simulink model "consensus_swarm_3"  (R2026a)
settings: Solver=ode4  FixedStep=0.004
undefined symbols (not defined in the file or in its folder): consensus_swarm_step, controlParams, eQ, eT, GravityAcc, kQ, kT, Mass, minPWM, rotorsSpeedDown, rotorsSpeedUp, SampleTime, uavParam
libraries: slpidlib x72, simulink x33, robotcorelib x12, matrix_library x12, aerolibasang x12, aerolibobsolete x3, uavutilslib x3
(part 1 of 9)
settings Model: Creator=Aaron  LastModifiedBy=Aaron

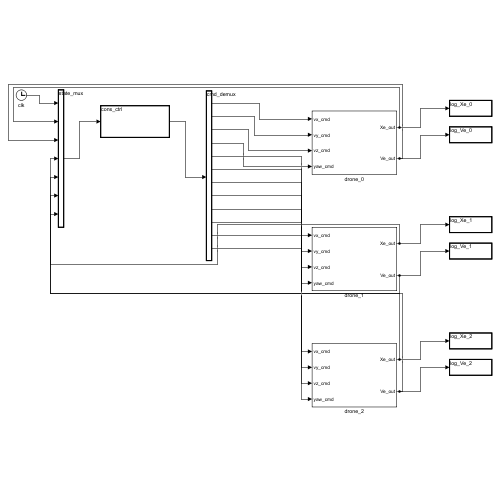
[thumbnail: Simulink's stored preview of the top-level diagram]
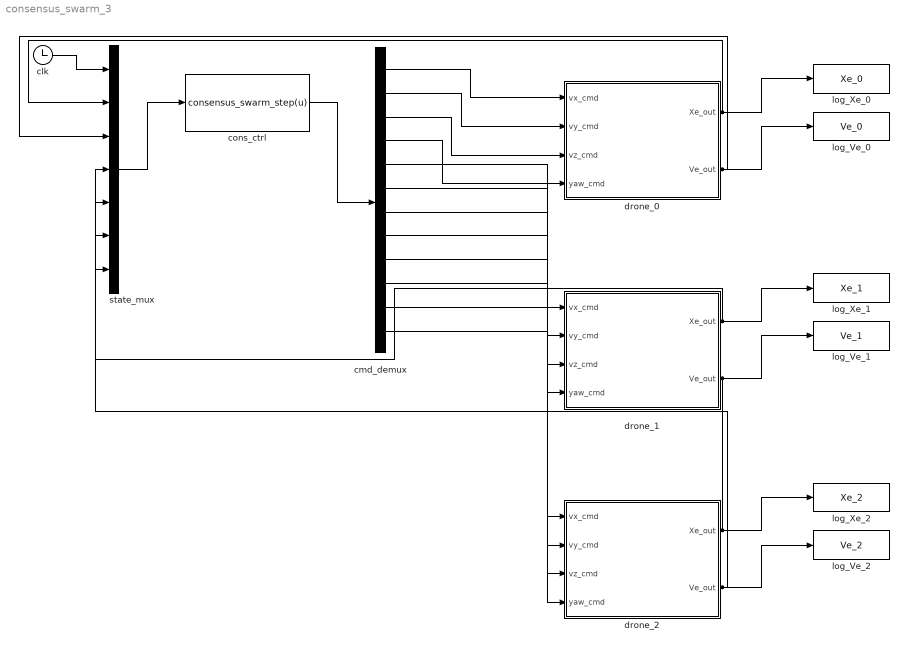
== system consensus_swarm_3 ==
  clk : Clock
  cmd_demux : Demux  Outputs=12
  cons_ctrl : MATLABFcn  MATLABFcn=consensus_swarm_step(u)  OutputDimensions=12  SampleTime=0.02
  drone_0 : Subsystem
  drone_1 : Subsystem
  drone_2 : Subsystem
  log_Ve_0 : ToWorkspace  VariableName=Ve_0  SaveFormat=Timeseries  SampleTime=-1
  log_Ve_1 : ToWorkspace  VariableName=Ve_1  SaveFormat=Timeseries  SampleTime=-1
  log_Ve_2 : ToWorkspace  VariableName=Ve_2  SaveFormat=Timeseries  SampleTime=-1
  log_Xe_0 : ToWorkspace  VariableName=Xe_0  SaveFormat=Timeseries  SampleTime=-1
  log_Xe_1 : ToWorkspace  VariableName=Xe_1  SaveFormat=Timeseries  SampleTime=-1
  log_Xe_2 : ToWorkspace  VariableName=Xe_2  SaveFormat=Timeseries  SampleTime=-1
  state_mux : Mux  Inputs=7
  wires:
  clk/1 -> state_mux/1
  state_mux/1 -> cons_ctrl/1
  cons_ctrl/1 -> cmd_demux/1
  drone_0/1(Xe_out) -> state_mux/2, log_Xe_0/1
  drone_0/2(Ve_out) -> state_mux/3, log_Ve_0/1
  cmd_demux/1 -> drone_0/1(vx_cmd)
  cmd_demux/2 -> drone_0/2(vy_cmd)
  cmd_demux/3 -> drone_0/3(vz_cmd)
  cmd_demux/4 -> drone_0/4(yaw_cmd)
  drone_1/1(Xe_out) -> state_mux/4, log_Xe_1/1
  drone_1/2(Ve_out) -> state_mux/5, log_Ve_1/1
  cmd_demux/5 -> drone_1/1(vx_cmd)
  cmd_demux/6 -> drone_1/2(vy_cmd)
  cmd_demux/7 -> drone_1/3(vz_cmd)
  cmd_demux/8 -> drone_1/4(yaw_cmd)
  drone_2/1(Xe_out) -> state_mux/6, log_Xe_2/1
  drone_2/2(Ve_out) -> state_mux/7, log_Ve_2/1
  cmd_demux/9 -> drone_2/1(vx_cmd)
  cmd_demux/10 -> drone_2/2(vy_cmd)
  cmd_demux/11 -> drone_2/3(vz_cmd)
  cmd_demux/12 -> drone_2/4(yaw_cmd)

== system consensus_swarm_3/drone_0 ==
  vx_cmd : Inport
  vy_cmd : Inport  Port=2
  vz_cmd : Inport  Port=3
  yaw_cmd : Inport  Port=4
  6DOF (Euler Angles) : aerolibobsolete/6DOF (Euler Angles)  units=Metric (MKS)  mtype=Fixed  rep=Euler Angles  xme_0=[0, 0, 0]  Vm_0=[0 0 0]  eul_0=[0 0 0]  pm_0=[0 0 0]  mass_0=Mass  mass_e=0.5  mass_f=2.0  inertia=momentInertia  inertia_e=eye(3)  inertia_f=2*eye(3)  k_quat=1.0  vre_flag=on  abi_flag=on  aMode=0  xme_statename=''  Vm_statename=''  eul_statename=''  quat_statename=''  pm_statename=''  mass_statename=''
  Add : Sum
  Bus Creator : BusCreator  Inputs=4
  Display17 : Display
  Gravity : Subsystem
  Mux4 : Mux  Inputs=3
  Selector1 : Selector  InputPortWidth=3  IndexOptions=Index vector (dialog)  Indices=[3 2 1]  OutputSizes=1
  Step4 : Step  Time=5  SampleTime=0
  Subsystem : Subsystem
  UAV Animation : uavutilslib/UAV Animation  Commented=on  NumUAV=1  DynamicUAVConfig=off  UAVType=Multirotor  UAVSize=5  UAVColor=[1 0 0]  UAVTrajectoryAlpha=1  AlwaysShowAnimation=on  AxisLimits=[-Inf Inf;-Inf Inf;-Inf Inf]  TrajectoryBufferSize=100000  InertialZDirection=Down  RotationFormat=Euler ZYX  DrawMarkers=off  SampleTime=-1
  pid_velocity : Subsystem
  z : Constant  Value=0
  Xe_out : Outport
  Ve_out : Outport  Port=2
  wires:
  Mux4/1 -> pid_velocity/2(vxyz_d)  "vel_cmd"
  z/1 -> ?
  [States] -> pid_velocity/1(estStates)
  pid_velocity/1(acts_w) -> Display17/1, [pid_pos]  "pid"
  [pid_pos] -> Subsystem/1(actCmd)
  Add/1 -> 6DOF (Euler Angles)/1
  Subsystem/1(F) -> Add/1
  Gravity/1(F_g) -> Add/2  "Gravity Force"
  Subsystem/2(M) -> 6DOF (Euler Angles)/2
  Bus Creator/1 -> [States]
  6DOF (Euler Angles)/4 -> [DCMbe]  "DCMbe"
  [DCMbe] -> Gravity/1(DCM_be)
  6DOF (Euler Angles)/1 -> Ve_out/1, [Ve]  "Ve"
  [Ve] -> Bus Creator/1
  [Xe] -> Bus Creator/2
  6DOF (Euler Angles)/3 -> [Euler], Selector1/1  "Euler"
  [Euler] -> Bus Creator/3
  6DOF (Euler Angles)/6 -> [pqr]  "pqr"
  [pqr] -> Bus Creator/4
  6DOF (Euler Angles)/2 -> Xe_out/1, [Xe], UAV Animation/1  "Xe"
  Selector1/1 -> UAV Animation/2
  vx_cmd/1 -> Mux4/1
  vy_cmd/1 -> Mux4/2
  vz_cmd/1 -> Mux4/3
  yaw_cmd/1 -> [uav_plant_io_yaw_cmd]

== system consensus_swarm_3/drone_1 ==
  vx_cmd : Inport
  vy_cmd : Inport  Port=2
  vz_cmd : Inport  Port=3
  yaw_cmd : Inport  Port=4
  6DOF (Euler Angles) : aerolibobsolete/6DOF (Euler Angles)  units=Metric (MKS)  mtype=Fixed  rep=Euler Angles  xme_0=[0, 0, 0]  Vm_0=[0 0 0]  eul_0=[0 0 0]  pm_0=[0 0 0]  mass_0=Mass  mass_e=0.5  mass_f=2.0  inertia=momentInertia  inertia_e=eye(3)  inertia_f=2*eye(3)  k_quat=1.0  vre_flag=on  abi_flag=on  aMode=0  xme_statename=''  Vm_statename=''  eul_statename=''  quat_statename=''  pm_statename=''  mass_statename=''
  Add : Sum
  Bus Creator : BusCreator  Inputs=4
  Display17 : Display
  Gravity : Subsystem
  Mux4 : Mux  Inputs=3
  Selector1 : Selector  InputPortWidth=3  IndexOptions=Index vector (dialog)  Indices=[3 2 1]  OutputSizes=1
  Step4 : Step  Time=5  SampleTime=0
  Subsystem : Subsystem
  UAV Animation : uavutilslib/UAV Animation  Commented=on  NumUAV=1  DynamicUAVConfig=off  UAVType=Multirotor  UAVSize=5  UAVColor=[1 0 0]  UAVTrajectoryAlpha=1  AlwaysShowAnimation=on  AxisLimits=[-Inf Inf;-Inf Inf;-Inf Inf]  TrajectoryBufferSize=100000  InertialZDirection=Down  RotationFormat=Euler ZYX  DrawMarkers=off  SampleTime=-1
  pid_velocity : Subsystem
  z : Constant  Value=0
  Xe_out : Outport
  Ve_out : Outport  Port=2
  wires:
  Mux4/1 -> pid_velocity/2(vxyz_d)  "vel_cmd"
  z/1 -> ?
  [States] -> pid_velocity/1(estStates)
  pid_velocity/1(acts_w) -> Display17/1, [pid_pos]  "pid"
  [pid_pos] -> Subsystem/1(actCmd)
  Add/1 -> 6DOF (Euler Angles)/1
  Subsystem/1(F) -> Add/1
  Gravity/1(F_g) -> Add/2  "Gravity Force"
  Subsystem/2(M) -> 6DOF (Euler Angles)/2
  Bus Creator/1 -> [States]
  6DOF (Euler Angles)/4 -> [DCMbe]  "DCMbe"
  [DCMbe] -> Gravity/1(DCM_be)
  6DOF (Euler Angles)/1 -> Ve_out/1, [Ve]  "Ve"
  [Ve] -> Bus Creator/1
  [Xe] -> Bus Creator/2
  6DOF (Euler Angles)/3 -> [Euler], Selector1/1  "Euler"
  [Euler] -> Bus Creator/3
  6DOF (Euler Angles)/6 -> [pqr]  "pqr"
  [pqr] -> Bus Creator/4
  6DOF (Euler Angles)/2 -> Xe_out/1, [Xe], UAV Animation/1  "Xe"
  Selector1/1 -> UAV Animation/2
  vx_cmd/1 -> Mux4/1
  vy_cmd/1 -> Mux4/2
  vz_cmd/1 -> Mux4/3
  yaw_cmd/1 -> [uav_plant_io_yaw_cmd]

== system consensus_swarm_3/drone_2 ==
  vx_cmd : Inport
  vy_cmd : Inport  Port=2
  vz_cmd : Inport  Port=3
  yaw_cmd : Inport  Port=4
  6DOF (Euler Angles) : aerolibobsolete/6DOF (Euler Angles)  units=Metric (MKS)  mtype=Fixed  rep=Euler Angles  xme_0=[0, 0, 0]  Vm_0=[0 0 0]  eul_0=[0 0 0]  pm_0=[0 0 0]  mass_0=Mass  mass_e=0.5  mass_f=2.0  inertia=momentInertia  inertia_e=eye(3)  inertia_f=2*eye(3)  k_quat=1.0  vre_flag=on  abi_flag=on  aMode=0  xme_statename=''  Vm_statename=''  eul_statename=''  quat_statename=''  pm_statename=''  mass_statename=''
  Add : Sum
  Bus Creator : BusCreator  Inputs=4
  Display17 : Display
  Gravity : Subsystem
  Mux4 : Mux  Inputs=3
  Selector1 : Selector  InputPortWidth=3  IndexOptions=Index vector (dialog)  Indices=[3 2 1]  OutputSizes=1
  Step4 : Step  Time=5  SampleTime=0
  Subsystem : Subsystem
  UAV Animation : uavutilslib/UAV Animation  Commented=on  NumUAV=1  DynamicUAVConfig=off  UAVType=Multirotor  UAVSize=5  UAVColor=[1 0 0]  UAVTrajectoryAlpha=1  AlwaysShowAnimation=on  AxisLimits=[-Inf Inf;-Inf Inf;-Inf Inf]  TrajectoryBufferSize=100000  InertialZDirection=Down  RotationFormat=Euler ZYX  DrawMarkers=off  SampleTime=-1
  pid_velocity : Subsystem
  z : Constant  Value=0
  Xe_out : Outport
  Ve_out : Outport  Port=2
  wires:
  Mux4/1 -> pid_velocity/2(vxyz_d)  "vel_cmd"
  z/1 -> ?
  [States] -> pid_velocity/1(estStates)
  pid_velocity/1(acts_w) -> Display17/1, [pid_pos]  "pid"
  [pid_pos] -> Subsystem/1(actCmd)
  Add/1 -> 6DOF (Euler Angles)/1
  Subsystem/1(F) -> Add/1
  Gravity/1(F_g) -> Add/2  "Gravity Force"
  Subsystem/2(M) -> 6DOF (Euler Angles)/2
  Bus Creator/1 -> [States]
  6DOF (Euler Angles)/4 -> [DCMbe]  "DCMbe"
  [DCMbe] -> Gravity/1(DCM_be)
  6DOF (Euler Angles)/1 -> Ve_out/1, [Ve]  "Ve"
  [Ve] -> Bus Creator/1
  [Xe] -> Bus Creator/2
  6DOF (Euler Angles)/3 -> [Euler], Selector1/1  "Euler"
  [Euler] -> Bus Creator/3
  6DOF (Euler Angles)/6 -> [pqr]  "pqr"
  [pqr] -> Bus Creator/4
  6DOF (Euler Angles)/2 -> Xe_out/1, [Xe], UAV Animation/1  "Xe"
  Selector1/1 -> UAV Animation/2
  vx_cmd/1 -> Mux4/1
  vy_cmd/1 -> Mux4/2
  vz_cmd/1 -> Mux4/3
  yaw_cmd/1 -> [uav_plant_io_yaw_cmd]

== system consensus_swarm_3/drone_0/Gravity ==
  DCM_be : Inport
  Constant : Constant  Value=[0 0 GravityAcc]'
  Display4 : Display
  Gain : Gain  Gain=Mass
  Matrix Multiply : Product  Multiplication=Matrix(*)
  F_g : Outport
  wires:
  Gain/1 -> F_g/1, Display4/1
  DCM_be/1 -> Matrix Multiply/1
  Constant/1 -> Matrix Multiply/2
  Matrix Multiply/1 -> Gain/1

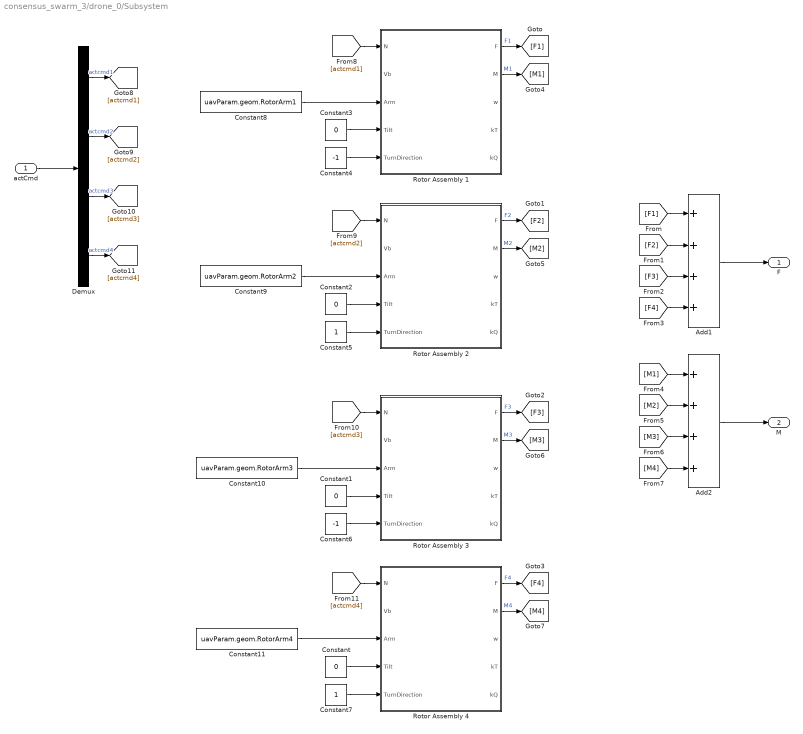
== system consensus_swarm_3/drone_0/Subsystem ==
  actCmd : Inport
  Add1 : Sum  Inputs=++++
  Add2 : Sum  Inputs=++++
  Constant{,1..3} (4 alike) : Constant  Value=0
  Constant10 : Constant  Value=uavParam.geom.RotorArm3
  Constant11 : Constant  Value=uavParam.geom.RotorArm4
  Constant4 : Constant  Value=-1
  Constant5 : Constant
  Constant6 : Constant  Value=-1
  Constant7 : Constant
  Constant8 : Constant  Value=uavParam.geom.RotorArm1
  Constant9 : Constant  Value=uavParam.geom.RotorArm2
  Demux : Demux
  Rotor Assembly 1 : Subsystem
  Rotor Assembly 2 : Subsystem
  Rotor Assembly 3 : Subsystem
  Rotor Assembly 4 : Subsystem
  F : Outport
  M : Outport  Port=2
  wires:
  [actcmd4] -> Rotor Assembly 4/1(N)
  Demux/4 -> [actcmd4]  "actcmd4"
  [actcmd3] -> Rotor Assembly 3/1(N)
  Demux/3 -> [actcmd3]  "actcmd3"
  [actcmd2] -> Rotor Assembly 2/1(N)
  Demux/2 -> [actcmd2]  "actcmd2"
  [actcmd1] -> Rotor Assembly 1/1(N)
  Demux/1 -> [actcmd1]  "actcmd1"
  actCmd/1 -> Demux/1
  [M4] -> Add2/4
  Rotor Assembly 4/2(M) -> [M4]  "M4"
  [M3] -> Add2/3
  Rotor Assembly 3/2(M) -> [M3]  "M3"
  [M2] -> Add2/2
  Rotor Assembly 2/2(M) -> [M2]  "M2"
  [M1] -> Add2/1
  Rotor Assembly 1/2(M) -> [M1]  "M1"
  [F4] -> Add1/4
  Rotor Assembly 4/1(F) -> [F4]  "F4"
  [F3] -> Add1/3
  Rotor Assembly 3/1(F) -> [F3]  "F3"
  [F2] -> Add1/2
  Rotor Assembly 2/1(F) -> [F2]  "F2"
  [F1] -> Add1/1
  Rotor Assembly 1/1(F) -> [F1]  "F1"
  Constant11/1 -> Rotor Assembly 4/3(Arm)
  Constant9/1 -> Rotor Assembly 2/3(Arm)
  Constant8/1 -> Rotor Assembly 1/3(Arm)
  Constant7/1 -> Rotor Assembly 4/5(TurnDirection)
  Constant5/1 -> Rotor Assembly 2/5(TurnDirection)
  Constant4/1 -> Rotor Assembly 1/5(TurnDirection)
  Constant3/1 -> Rotor Assembly 1/4(Tilt)
  Constant2/1 -> Rotor Assembly 2/4(Tilt)
  Constant/1 -> Rotor Assembly 4/4(Tilt)
  Add2/1 -> M/1
  Constant1/1 -> Rotor Assembly 3/4(Tilt)
  Constant6/1 -> Rotor Assembly 3/5(TurnDirection)
  ? -> Rotor Assembly 3/2(Vb)
  Add1/1 -> F/1
  Constant10/1 -> Rotor Assembly 3/3(Arm)

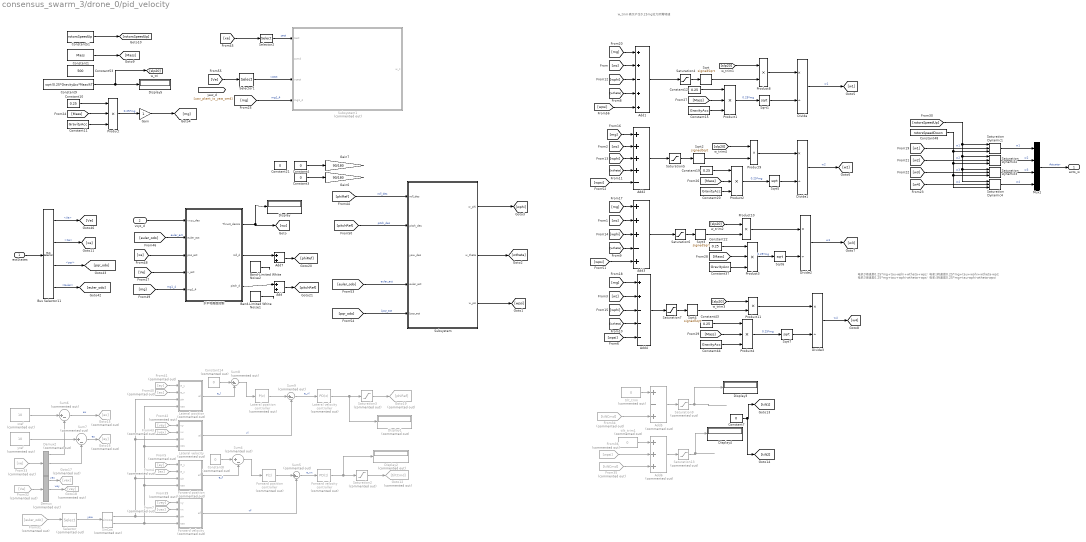
== system consensus_swarm_3/drone_0/pid_velocity ==
  note: w_trim 表示产生0.25mg拉力所需转速
  note: 电机1转速是0.25*mg+tau-wphi+wtheta+wpsi，
      | 电机2转速是0.25*mg+tau+wphi+wtheta-wpsi，
      | 电机3转速是0.25*mg+tau+wphi-wtheta+wpsi，
      | 电机4转速是0.25*mg+tau-wphi-wtheta-wpsi
  estStates : Inport
  vxyz_d : Inport  Port=2
  Add : Sum
  Add1 : Sum  Inputs=++-++
  Add2 : Sum  Inputs=++++-
  Add3 : Sum  Inputs=+++-+
  Add4 : Sum  Inputs=++---
  Add5 : Sum  Commented=on  Inputs=+-+
  Add6 : Sum  Commented=on  Inputs=+++
  Add7 : Sum
  Band-Limited White Noise1 : simulink/Sources/Band-Limited White Noise  Cov=[0.000001]  Ts=SampleTime  seed=[23341]
  Band-Limited White Noise2 : simulink/Sources/Band-Limited White Noise  Cov=[0.000001]  Ts=SampleTime  seed=[2341]
  Bus Selector11 : BusSelector  OutputSignals=Ve,Xe,pqr,Euler
  Constant1 : Constant  Value=Mass  OutDataTypeStr=double
  Constant{10,12,19,22,43} (5 alike) : Constant  Value=0.25  OutDataTypeStr=double
  Constant{11,15,20,37,44} (5 alike) : Constant  Value=GravityAcc  OutDataTypeStr=double
  Constant14 : Constant  Commented=on  Value=0
  Constant{3..4,7,21} (4 alike) : Constant  Value=0  OutDataTypeStr=double
  Constant48 : Constant  Value=rotorsSpeedDown  OutDataTypeStr=double
  Constant51 : Constant  Value=rotorsSpeedUp  OutDataTypeStr=double
  Constant53 : Constant  Value=500
  Constant8 : Constant  Commented=on  Value=0
  Constant9 : Constant  Value=sqrt(0.25*GravityAcc*Mass/kT)
  Demux : Demux  Commented=on  Outputs=3
  Demux2 : Demux  Commented=on  Outputs=3
  Display{,3..5} (4 alike) : Display
  Display1 : Display  Commented=on
  Display2 : Display  Commented=on
  Divide{,1..3} (4 alike) : Product  Inputs=*/
  Forward position : Subsystem  Commented=on
  Forward position controller : slpidlib/PID Controller  Commented=on  Controller=P  Form=Parallel  TimeDomain=Discrete-time  UseExternalTs=off  SampleTime=-1  IntegratorMethod=Forward Euler  FilterMethod=Forward Euler  ControllerParametersSource=internal  P=1  I=controlParams.I_X  UseKiTs=off  D=0.741088334151374  UseExternalDerivativeSource=off  N=1.14081860742283  UseFilter=on  TunerSelectOption=Transfer Function Based (PID Tuner App)  InitialConditionSource=internal  InitialConditionForIntegrator=0  InitialConditionForFilter=0  DifferentiatorICPrevScaledInput=0  ExternalReset=none  TrackingMode=off  Kt=1  LimitOutput=off  SatLimitsSource=internal  UpperSaturationLimit=inf  LowerSaturationLimit=-inf  LinearizeAsGain=on  AntiWindupMode=none  Kb=1  LimitIntegrator=off  UpperIntegratorSaturationLimit=inf  LowerIntegratorSaturationLimit=-inf  POutMin=[]  POutMax=[]  IOutMin=[]  IOutMax=[]  DOutMin=[]  DOutMax=[]  NOutMin=[]  NOutMax=[]  SumOutMin=[]  SumOutMax=[]  SaturationOutMin=[]  SaturationOutMax=[]  PParamMin=[]  PParamMax=[]  IParamMin=[]  IParamMax=[]  DParamMin=[]  DParamMax=[]  NParamMin=[]  NParamMax=[]  KbParamMin=[]  KbParamMax=[]  KtParamMin=[]  KtParamMax=[]  KbOutMin=[]  KbOutMax=[]  KtOutMin=[]  KtOutMax=[]  IntegratorOutMin=[]  IntegratorOutMax=[]  FilterOutMin=[]  FilterOutMax=[]  SumI1OutMin=[]  SumI1OutMax=[]  SumI2OutMin=[]  SumI2OutMax=[]  SumI3OutMin=[]  SumI3OutMax=[]  SumI4OutMin=[]  SumI4OutMax=[]  SumDOutMin=[]  SumDOutMax=[]  DifferentiatorOutMin=[]  DifferentiatorOutMax=[]  FilterDiffOutCoefMin=[]  FilterDiffOutCoefMax=[]  ReciprocalOutMin=[]  ReciprocalOutMax=[]  SumDenOutMin=[]  SumDenOutMax=[]  SumNumOutMin=[]  SumNumOutMax=[]  DivideOutMin=[]  DivideOutMax=[]  UdiffTsProdOutMin=[]  UdiffTsProdOutMax=[]  NTsProdOutMin=[]  NTsProdOutMax=[]  UintegralTsProdOutMin=[]  UintegralTsProdOutMax=[]  UngainTsProdOutMin=[]  UngainTsProdOutMax=[]  ClampingZeroOutDataTypeStr=Inherit: Inherit via back propagation  ClampingZeroOutMin=[]  ClampingZeroOutMax=[]  FilterDenConstantOutDataTypeStr=Inherit: Inherit via back propagation  FilterDenConstantOutMin=[]  FilterDenConstantOutMax=[]  PCopyOutDataTypeStr=Inherit: Inherit via back propagation  PCopyOutMin=[]  PCopyOutMax=[]  NCopyOutDataTypeStr=Inherit: Inherit via back propagation  NCopyOutMin=[]  NCopyOutMax=[]  IntegratorContinuousStateAttributes=''  IntegratorStateMustResolveToSignalObject=off  IntegratorRTWStateStorageClass=Auto  FilterContinuousStateAttributes=''  FilterStateMustResolveToSignalObject=off  FilterRTWStateStorageClass=Auto  ParallelPVariant=InternalParameters  IdealPVariant=Disabled  IVariant=Disabled  DVariant=Disabled  IntegratorVariant=Disabled  SatVariant=Disabled  AWVariant=Disabled  PCopyVariant=Disabled  TRVariant=Disabled  FdbkBlocksVariant=Forward  IdealPFdbkVariant=Disabled  SatFdbkVariant=Disabled  DerivativeFilterVariant=Disabled  NVariant=Disabled  NCopyVariant=Disabled_SignalSpec  FilterICVariant=Disabled  IntegratorICVariant=Disabled  ExternalResetVariant=Disabled  TRSumVariant=Passthrough  SumFdbkVariant=Disabled  SumVariant=Passthrough_P  TsampFilterVariant=InternalTs  TsampNgainVariant=Passthrough  TsampIntegralVariant=Disabled_SignalSpec  ExternalSaturationOutDataTypeStr=Inherit: Same as second input  DerivativeSourceVariant=Disabled  PreIntVariant=InternalPreInt
  Forward velocity : Subsystem  Commented=on
  Forward velocity controller : slpidlib/PID Controller  Commented=on  Controller=PD  Form=Parallel  TimeDomain=Discrete-time  UseExternalTs=off  SampleTime=-1  IntegratorMethod=Forward Euler  FilterMethod=Forward Euler  ControllerParametersSource=internal  P=10  I=0  UseKiTs=off  D=0.1  UseExternalDerivativeSource=off  N=20  UseFilter=on  TunerSelectOption=Transfer Function Based (PID Tuner App)  InitialConditionSource=internal  InitialConditionForIntegrator=0  InitialConditionForFilter=0  DifferentiatorICPrevScaledInput=0  ExternalReset=none  TrackingMode=off  Kt=1  LimitOutput=off  SatLimitsSource=internal  UpperSaturationLimit=inf  LowerSaturationLimit=-inf  LinearizeAsGain=on  AntiWindupMode=none  Kb=1  LimitIntegrator=off  UpperIntegratorSaturationLimit=inf  LowerIntegratorSaturationLimit=-inf  POutMin=[]  POutMax=[]  IOutMin=[]  IOutMax=[]  DOutMin=[]  DOutMax=[]  NOutMin=[]  NOutMax=[]  SumOutMin=[]  SumOutMax=[]  SaturationOutMin=[]  SaturationOutMax=[]  PParamMin=[]  PParamMax=[]  IParamMin=[]  IParamMax=[]  DParamMin=[]  DParamMax=[]  NParamMin=[]  NParamMax=[]  KbParamMin=[]  KbParamMax=[]  KtParamMin=[]  KtParamMax=[]  KbOutMin=[]  KbOutMax=[]  KtOutMin=[]  KtOutMax=[]  IntegratorOutMin=[]  IntegratorOutMax=[]  FilterOutMin=[]  FilterOutMax=[]  SumI1OutMin=[]  SumI1OutMax=[]  SumI2OutMin=[]  SumI2OutMax=[]  SumI3OutMin=[]  SumI3OutMax=[]  SumI4OutMin=[]  SumI4OutMax=[]  SumDOutMin=[]  SumDOutMax=[]  DifferentiatorOutMin=[]  DifferentiatorOutMax=[]  FilterDiffOutCoefMin=[]  FilterDiffOutCoefMax=[]  ReciprocalOutMin=[]  ReciprocalOutMax=[]  SumDenOutMin=[]  SumDenOutMax=[]  SumNumOutMin=[]  SumNumOutMax=[]  DivideOutMin=[]  DivideOutMax=[]  UdiffTsProdOutMin=[]  UdiffTsProdOutMax=[]  NTsProdOutMin=[]  NTsProdOutMax=[]  UintegralTsProdOutMin=[]  UintegralTsProdOutMax=[]  UngainTsProdOutMin=[]  UngainTsProdOutMax=[]  ClampingZeroOutDataTypeStr=Inherit: Inherit via back propagation  ClampingZeroOutMin=[]  ClampingZeroOutMax=[]  FilterDenConstantOutDataTypeStr=Inherit: Inherit via back propagation  FilterDenConstantOutMin=[]  FilterDenConstantOutMax=[]  PCopyOutDataTypeStr=Inherit: Inherit via back propagation  PCopyOutMin=[]  PCopyOutMax=[]  NCopyOutDataTypeStr=Inherit: Inherit via back propagation  NCopyOutMin=[]  NCopyOutMax=[]  IntegratorContinuousStateAttributes=''  IntegratorStateMustResolveToSignalObject=off  IntegratorRTWStateStorageClass=Auto  FilterContinuousStateAttributes=''  FilterStateMustResolveToSignalObject=off  FilterRTWStateStorageClass=Auto  ParallelPVariant=InternalParameters  IdealPVariant=Disabled  IVariant=Disabled  DVariant=InternalParameters  IntegratorVariant=Disabled  SatVariant=Disabled  AWVariant=Disabled  PCopyVariant=Disabled  TRVariant=Disabled  FdbkBlocksVariant=Forward  IdealPFdbkVariant=Disabled  SatFdbkVariant=Disabled  DerivativeFilterVariant=ForwardEulerFilter  NVariant=InternalParameters  NCopyVariant=Disabled  FilterICVariant=InternalICsFilter  IntegratorICVariant=Disabled  ExternalResetVariant=Disabled  TRSumVariant=Passthrough  SumFdbkVariant=Disabled  SumVariant=Sum_PD  TsampFilterVariant=InternalTs  TsampNgainVariant=Passthrough  TsampIntegralVariant=Disabled_SignalSpec  ExternalSaturationOutDataTypeStr=Inherit: Same as second input  DerivativeSourceVariant=ErrorSignal  PreIntVariant=InternalPreInt
  From31 : From  Commented=on  GotoTag=euler_odo
  From32 : From  Commented=on  GotoTag=Ve
  From33 : From  Commented=on  GotoTag=xe
  From34 : From  Commented=on  GotoTag=tiltCmd
  From35 : From  Commented=on  GotoTag=tiltCmd
  From36 : From  Commented=on  GotoTag=wpsi
  From39 : From  Commented=on  GotoTag=vey
  From4 : From  Commented=on  GotoTag=ex
  From40 : From  Commented=on  GotoTag=ex
  From41 : From  Commented=on  GotoTag=ey
  From42 : From  Commented=on  GotoTag=vey
  From43 : From  Commented=on  GotoTag=vex
  From5 : From  Commented=on  GotoTag=ey
  From7 : From  Commented=on  GotoTag=vex
  Gain : Gain
  Gain6 : Gain  Gain=90/180
  Gain7 : Gain  Gain=90/180
  Goto12 : Goto  Commented=on  GotoTag=tiltCmd
  Goto15 : Goto  Commented=on  GotoTag=ex
  Goto16 : Goto  Commented=on  GotoTag=ey
  Goto17 : Goto  Commented=on  GotoTag=vex
  Goto18 : Goto  Commented=on  GotoTag=vey
  Goto19 : Goto  Commented=on  GotoTag=phiRef
  Lateral position : Subsystem  Commented=on
  Lateral position controller : slpidlib/PID Controller  Commented=on  Controller=P  Form=Parallel  TimeDomain=Discrete-time  UseExternalTs=off  SampleTime=-1  IntegratorMethod=Forward Euler  FilterMethod=Forward Euler  ControllerParametersSource=internal  P=1  I=controlParams.I_Y  UseKiTs=off  D=0.20966837124708  UseExternalDerivativeSource=off  N=1.18305565097938  UseFilter=on  TunerSelectOption=Transfer Function Based (PID Tuner App)  InitialConditionSource=internal  InitialConditionForIntegrator=0  InitialConditionForFilter=0  DifferentiatorICPrevScaledInput=0  ExternalReset=none  TrackingMode=off  Kt=1  LimitOutput=off  SatLimitsSource=internal  UpperSaturationLimit=0.4  LowerSaturationLimit=-0.4  LinearizeAsGain=on  AntiWindupMode=clamping  Kb=1  LimitIntegrator=off  UpperIntegratorSaturationLimit=inf  LowerIntegratorSaturationLimit=-inf  POutMin=[]  POutMax=[]  IOutMin=[]  IOutMax=[]  DOutMin=[]  DOutMax=[]  NOutMin=[]  NOutMax=[]  SumOutMin=[]  SumOutMax=[]  SaturationOutMin=[]  SaturationOutMax=[]  PParamMin=[]  PParamMax=[]  IParamMin=[]  IParamMax=[]  DParamMin=[]  DParamMax=[]  NParamMin=[]  NParamMax=[]  KbParamMin=[]  KbParamMax=[]  KtParamMin=[]  KtParamMax=[]  KbOutMin=[]  KbOutMax=[]  KtOutMin=[]  KtOutMax=[]  IntegratorOutMin=[]  IntegratorOutMax=[]  FilterOutMin=[]  FilterOutMax=[]  SumI1OutMin=[]  SumI1OutMax=[]  SumI2OutMin=[]  SumI2OutMax=[]  SumI3OutMin=[]  SumI3OutMax=[]  SumI4OutMin=[]  SumI4OutMax=[]  SumDOutMin=[]  SumDOutMax=[]  DifferentiatorOutMin=[]  DifferentiatorOutMax=[]  FilterDiffOutCoefMin=[]  FilterDiffOutCoefMax=[]  ReciprocalOutMin=[]  ReciprocalOutMax=[]  SumDenOutMin=[]  SumDenOutMax=[]  SumNumOutMin=[]  SumNumOutMax=[]  DivideOutMin=[]  DivideOutMax=[]  UdiffTsProdOutMin=[]  UdiffTsProdOutMax=[]  NTsProdOutMin=[]  NTsProdOutMax=[]  UintegralTsProdOutMin=[]  UintegralTsProdOutMax=[]  UngainTsProdOutMin=[]  UngainTsProdOutMax=[]  ClampingZeroOutDataTypeStr=Inherit: Inherit via back propagation  ClampingZeroOutMin=[]  ClampingZeroOutMax=[]  FilterDenConstantOutDataTypeStr=Inherit: Inherit via back propagation  FilterDenConstantOutMin=[]  FilterDenConstantOutMax=[]  PCopyOutDataTypeStr=Inherit: Inherit via back propagation  PCopyOutMin=[]  PCopyOutMax=[]  NCopyOutDataTypeStr=Inherit: Inherit via back propagation  NCopyOutMin=[]  NCopyOutMax=[]  IntegratorContinuousStateAttributes=''  IntegratorStateMustResolveToSignalObject=off  IntegratorRTWStateStorageClass=Auto  FilterContinuousStateAttributes=''  FilterStateMustResolveToSignalObject=off  FilterRTWStateStorageClass=Auto  ParallelPVariant=InternalParameters  IdealPVariant=Disabled  IVariant=Disabled  DVariant=Disabled  IntegratorVariant=Disabled  SatVariant=Disabled  AWVariant=Disabled  PCopyVariant=Disabled  TRVariant=Disabled  FdbkBlocksVariant=Forward  IdealPFdbkVariant=Disabled  SatFdbkVariant=Disabled  DerivativeFilterVariant=Disabled  NVariant=Disabled  NCopyVariant=Disabled_SignalSpec  FilterICVariant=Disabled  IntegratorICVariant=Disabled  ExternalResetVariant=Disabled  TRSumVariant=Passthrough  SumFdbkVariant=Disabled  SumVariant=Passthrough_P  TsampFilterVariant=InternalTs  TsampNgainVariant=Passthrough  TsampIntegralVariant=Disabled_SignalSpec  ExternalSaturationOutDataTypeStr=Inherit: Same as second input  DerivativeSourceVariant=Disabled  PreIntVariant=InternalPreInt
  Lateral velocity : Subsystem  Commented=on
  "Lateral velocity controller " : slpidlib/PID Controller  Commented=on  Controller=PD  Form=Parallel  TimeDomain=Discrete-time  UseExternalTs=off  SampleTime=-1  IntegratorMethod=Forward Euler  FilterMethod=Forward Euler  ControllerParametersSource=internal  P=10  I=0  UseKiTs=off  D=0.1  UseExternalDerivativeSource=off  N=20  UseFilter=on  TunerSelectOption=Transfer Function Based (PID Tuner App)  InitialConditionSource=internal  InitialConditionForIntegrator=0  InitialConditionForFilter=0  DifferentiatorICPrevScaledInput=0  ExternalReset=none  TrackingMode=off  Kt=1  LimitOutput=off  SatLimitsSource=internal  UpperSaturationLimit=inf  LowerSaturationLimit=-inf  LinearizeAsGain=on  AntiWindupMode=none  Kb=1  LimitIntegrator=off  UpperIntegratorSaturationLimit=inf  LowerIntegratorSaturationLimit=-inf  POutMin=[]  POutMax=[]  IOutMin=[]  IOutMax=[]  DOutMin=[]  DOutMax=[]  NOutMin=[]  NOutMax=[]  SumOutMin=[]  SumOutMax=[]  SaturationOutMin=[]  SaturationOutMax=[]  PParamMin=[]  PParamMax=[]  IParamMin=[]  IParamMax=[]  DParamMin=[]  DParamMax=[]  NParamMin=[]  NParamMax=[]  KbParamMin=[]  KbParamMax=[]  KtParamMin=[]  KtParamMax=[]  KbOutMin=[]  KbOutMax=[]  KtOutMin=[]  KtOutMax=[]  IntegratorOutMin=[]  IntegratorOutMax=[]  FilterOutMin=[]  FilterOutMax=[]  SumI1OutMin=[]  SumI1OutMax=[]  SumI2OutMin=[]  SumI2OutMax=[]  SumI3OutMin=[]  SumI3OutMax=[]  SumI4OutMin=[]  SumI4OutMax=[]  SumDOutMin=[]  SumDOutMax=[]  DifferentiatorOutMin=[]  DifferentiatorOutMax=[]  FilterDiffOutCoefMin=[]  FilterDiffOutCoefMax=[]  ReciprocalOutMin=[]  ReciprocalOutMax=[]  SumDenOutMin=[]  SumDenOutMax=[]  SumNumOutMin=[]  SumNumOutMax=[]  DivideOutMin=[]  DivideOutMax=[]  UdiffTsProdOutMin=[]  UdiffTsProdOutMax=[]  NTsProdOutMin=[]  NTsProdOutMax=[]  UintegralTsProdOutMin=[]  UintegralTsProdOutMax=[]  UngainTsProdOutMin=[]  UngainTsProdOutMax=[]  ClampingZeroOutDataTypeStr=Inherit: Inherit via back propagation  ClampingZeroOutMin=[]  ClampingZeroOutMax=[]  FilterDenConstantOutDataTypeStr=Inherit: Inherit via back propagation  FilterDenConstantOutMin=[]  FilterDenConstantOutMax=[]  PCopyOutDataTypeStr=Inherit: Inherit via back propagation  PCopyOutMin=[]  PCopyOutMax=[]  NCopyOutDataTypeStr=Inherit: Inherit via back propagation  NCopyOutMin=[]  NCopyOutMax=[]  IntegratorContinuousStateAttributes=''  IntegratorStateMustResolveToSignalObject=off  IntegratorRTWStateStorageClass=Auto  FilterContinuousStateAttributes=''  FilterStateMustResolveToSignalObject=off  FilterRTWStateStorageClass=Auto  ParallelPVariant=InternalParameters  IdealPVariant=Disabled  IVariant=Disabled  DVariant=InternalParameters  IntegratorVariant=Disabled  SatVariant=Disabled  AWVariant=Disabled  PCopyVariant=Disabled  TRVariant=Disabled  FdbkBlocksVariant=Forward  IdealPFdbkVariant=Disabled  SatFdbkVariant=Disabled  DerivativeFilterVariant=ForwardEulerFilter  NVariant=InternalParameters  NCopyVariant=Disabled  FilterICVariant=InternalICsFilter  IntegratorICVariant=Disabled  ExternalResetVariant=Disabled  TRSumVariant=Passthrough  SumFdbkVariant=Disabled  SumVariant=Sum_PD  TsampFilterVariant=InternalTs  TsampNgainVariant=Passthrough  TsampIntegralVariant=Disabled_SignalSpec  ExternalSaturationOutDataTypeStr=Inherit: Same as second input  DerivativeSourceVariant=ErrorSignal  PreIntVariant=InternalPreInt
  Mux1 : Mux
  Product{,1..4} (5 alike) : Product  Inputs=3
  Product{8..11} (4 alike) : Product
  Saturation Dynamic{1..4} (4 alike) : simulink/Discontinuities/Saturation Dynamic  OutMin=[]  OutMax=[]  OutDataTypeStr=double  OutDataType=fixdt(1, 16)  OutScaling=2^-10  DoSatur=off
  Saturation13 : Saturate  Commented=on  UpperLimit=0.3  LowerLimit=0
  Saturation2 : Saturate  Commented=on  UpperLimit=0.75  LowerLimit=-0.75
  Saturation3 : Saturate  Commented=on  UpperLimit=0.75  LowerLimit=-0.75
  Saturation{4..7} (4 alike) : Saturate  UpperLimit=inf  LowerLimit=0
  Saturation9 : Saturate  Commented=on  UpperLimit=0.3  LowerLimit=0
  Selector : Selector  Commented=on  InputPortWidth=3  IndexOptions=Index vector (dialog)  Indices=[3]  OutputSizes=1
  Selector1 : Selector  InputPortWidth=3  IndexOptions=Index vector (dialog)  Indices=[3]  OutputSizes=1
  Selector2 : Selector  InputPortWidth=3  IndexOptions=Index vector (dialog)  Indices=[3]  OutputSizes=1
  SinCos : Trigonometry  Commented=on  Operator=sincos
  Sqrt{,2..4} (4 alike) : Sqrt  Operator=signedSqrt
  Sqrt{1,5..7} (4 alike) : Sqrt
  Subsystem : Subsystem
  Subsystem1 : Subsystem  Commented=on
  Sum{4..9} (6 alike) : Sum  Commented=on  Inputs=|+-
  tilt_trim : Constant  Commented=on  Value=0
  tilt_trim1 : Constant  Commented=on  Value=0
  xref : Constant  Commented=on  Value=10  OutDataTypeStr=boolean
  yref : Constant  Commented=on  Value=10  OutDataTypeStr=boolean
  水平和高度控制 : Subsystem
  acts_w : Outport
  wires:
  Saturation3/1 -> Goto19/1
  [xe] -> Selector2/1
  "Lateral velocity controller "/1 -> Display1/1, Saturation3/1
  From43/1 -> Lateral velocity/2(vx)
  From42/1 -> Lateral velocity/1(vy)
  From41/1 -> Lateral position/1(e_y)
  From40/1 -> Lateral position/2(e_x)
  From39/1 -> Forward velocity/1(vy)
  Demux/2 -> Goto18/1  "vey"
  From7/1 -> Forward velocity/2(vx)
  Demux/1 -> Goto17/1  "vex"
  From5/1 -> Forward position/1(e_y)
  Sum7/1 -> Goto16/1  "ey"
  From4/1 -> Forward position/2(e_x)
  Sum6/1 -> Goto15/1  "ex"
  Lateral velocity/1(el) -> Sum9/2  "vl"
  Lateral position controller/1 -> Sum9/1
  Sum9/1 -> "Lateral velocity controller "/1  "e_vl"
  Constant14/1 -> Sum8/1
  Lateral position/1(el) -> Sum8/2  "e_l"
  Sum8/1 -> Lateral position controller/1
  Add6/1 -> Saturation13/1
  Add5/1 -> Saturation9/1
  From34/1 -> Add5/3
  ? -> Add5/2
  tilt_trim/1 -> Add5/1
  From35/1 -> Add6/3
  Saturation13/1 -> Display4/1
  tilt_trim1/1 -> Add6/1
  From36/1 -> Add6/2
  Saturation9/1 -> Display3/1
  Saturation2/1 -> Goto12/1
  yref/1 -> Sum7/1
  xref/1 -> Sum6/1
  Demux2/2 -> Sum7/2
  Demux2/1 -> Sum6/2
  From33/1 -> Demux2/1
  From32/1 -> Demux/1
  From31/1 -> Selector/1
  SinCos/1 -> Forward position/3(sin), Lateral velocity/3(sin), Lateral position/3(sin), Forward velocity/3(sin)
  SinCos/2 -> Forward velocity/4(cos), Forward position/4(cos), Lateral position/4(cos), Lateral velocity/4(cos)
  Selector/1 -> SinCos/1  "yaw"
  Forward position controller/1 -> Sum5/1
  Forward velocity/1(ef) -> Sum5/2  "vf"
  Sum4/1 -> Forward position controller/1
  Constant8/1 -> Sum4/1
  Forward velocity controller/1 -> Saturation2/1, Display2/1
  Sum5/1 -> Forward velocity controller/1  "e_vx"
  Forward position/1(ef) -> Sum4/2  "e_f"
  Constant3/1 -> Gain6/1
  Constant4/1 -> Gain7/1
  Sqrt2/1 -> Product9/2
  Sqrt3/1 -> Product10/2
  Saturation7/1 -> Sqrt4/1
  Add1/1 -> Saturation4/1
  Sqrt4/1 -> Product11/2
  Add2/1 -> Saturation5/1
  Saturation5/1 -> Sqrt2/1
  Sqrt/1 -> Product8/2
  Add4/1 -> Saturation7/1
  Add3/1 -> Saturation6/1
  Saturation6/1 -> Sqrt3/1
  Saturation4/1 -> Sqrt/1
  [wz] -> Add1/2
  [wz] -> Add3/2
  [wz] -> Add2/2
  [wz] -> Add4/2
  [wpsi] -> Add3/5
  [wpsi] -> Add1/5
  [wpsi] -> Add4/5
  [wpsi] -> Add2/5
  [wtheta] -> Add1/4
  [wtheta] -> Add3/4
  [wtheta] -> Add4/4
  [wtheta] -> Add2/4
  [wphi] -> Add1/3
  [wphi] -> Add2/3
  [wphi] -> Add3/3
  [wphi] -> Add4/3
  Product/1 -> Gain/1  "0.25*mg"
  [mg] -> Add1/1
  [mg] -> Add3/1
  [mg] -> Add2/1
  [mg] -> Add4/1
  Divide/1 -> [w1]  "w1"
  Divide1/1 -> [w2]  "w2"
  Divide2/1 -> [w3]  "w3"
  Divide3/1 -> [w4]  "w4"
  [Ve] -> Selector1/1
  Saturation Dynamic1/1 -> Mux1/1  "w1"
  Saturation Dynamic2/1 -> Mux1/2  "w2"
  Saturation Dynamic3/1 -> Mux1/3  "w3"
  Saturation Dynamic4/1 -> Mux1/4  "w4"
  Constant10/1 -> Product/1
  [Mass] -> Product/2
  Constant11/1 -> Product/3
  Sqrt1/1 -> Divide/2
  Constant15/1 -> Product1/3
  [Mass] -> Product1/2
  Constant12/1 -> Product1/1
  Product1/1 -> Sqrt1/1  "0.25*mg"
  Product8/1 -> Divide/1
  Product9/1 -> Divide1/1
  Product2/1 -> Sqrt5/1  "0.25*mg"
  Constant19/1 -> Product2/1
  [Mass] -> Product2/2
  Constant20/1 -> Product2/3
  Sqrt5/1 -> Divide1/2
  Sqrt6/1 -> Divide2/2
  Constant37/1 -> Product3/3
  [Mass] -> Product3/2
  Constant22/1 -> Product3/1
  Product3/1 -> Sqrt6/1  "0.25*mg"
  Product10/1 -> Divide2/1
  Product11/1 -> Divide3/1
  Product4/1 -> Sqrt7/1  "0.25*mg"
  Constant43/1 -> Product4/1
  [Mass] -> Product4/2
  Constant44/1 -> Product4/3
  Sqrt7/1 -> Divide3/2
  [slp20] -> Product8/1
  [slp20] -> Product9/1
  [slp20] -> Product10/1
  [slp20] -> Product11/1
  Constant48/1 -> Saturation Dynamic3/3, Saturation Dynamic4/3, Saturation Dynamic2/3, Saturation Dynamic1/3
  [rotorsSpeedUp] -> Saturation Dynamic3/1, Saturation Dynamic4/1, Saturation Dynamic2/1, Saturation Dynamic1/1
  [w1] -> Saturation Dynamic1/2  "w1"
  [w3] -> Saturation Dynamic3/2  "w3"
  [w4] -> Saturation Dynamic4/2  "w4"
  [w2] -> Saturation Dynamic2/2  "w2"
  estStates/1 -> Bus Selector11/1
  Mux1/1 -> acts_w/1  "Actuator"
  Constant1/1 -> [Mass]
  Constant9/1 -> Display5/1, [slp20]
  Constant51/1 -> [rotorsSpeedUp]
  Bus Selector11/1 -> [Ve]  "<Ve>"
  Bus Selector11/2 -> [xe]  "<Xe>"
  Bus Selector11/3 -> [pqr_odo]  "<pqr>"
  Bus Selector11/4 -> [euler_odo]  "<Euler>"
  [phiRef] -> Subsystem/1(roll_des)  "roll_des"
  [pitchRef] -> Subsystem/2(pitch_des)  "pitch_des"
  [euler_odo] -> Subsystem/4(euler_act)  "euler_act"
  [pqr_odo] -> Subsystem/5("[pqr_act")  "[pqr_act"
  Subsystem/1(w_phi) -> [wphi]
  Subsystem/2(w_theta) -> [wtheta]
  Subsystem/3(w_psi) -> [wpsi]
  [euler_odo] -> 水平和高度控制/2(euler_act)  "euler_act"
  [Ve] -> 水平和高度控制/4(v_act)
  [xe] -> 水平和高度控制/3(pos_act)
  水平和高度控制/2(roll_d) -> Add7/1
  vxyz_d/1 -> 水平和高度控制/1(vxyz_des)
  水平和高度控制/1(Thrust_desire) -> Display/1, [wz]
  Selector2/1 -> Subsystem1/1(zact)  "zact"
  ? -> Subsystem1/2(zcmd)  "zcmd"
  Selector1/1 -> Subsystem1/3(vzact)  "vzact"
  [mg] -> Subsystem1/4(mg1_4)  "mg1_4"
  [mg] -> 水平和高度控制/5(mg1_4)  "mg1_4"
  水平和高度控制/3(pitch_d) -> Add/1
  Constant7/1 -> [tilt2], [tilt1]
  Gain/1 -> [mg]
  Add/1 -> [pitchRef]
  Band-Limited White Noise1/1 -> ?
  Band-Limited White Noise2/1 -> ?
  Add7/1 -> [phiRef]

== system consensus_swarm_3/drone_1/Gravity ==
  DCM_be : Inport
  Constant : Constant  Value=[0 0 GravityAcc]'
  Display4 : Display
  Gain : Gain  Gain=Mass
  Matrix Multiply : Product  Multiplication=Matrix(*)
  F_g : Outport
  wires:
  Gain/1 -> F_g/1, Display4/1
  DCM_be/1 -> Matrix Multiply/1
  Constant/1 -> Matrix Multiply/2
  Matrix Multiply/1 -> Gain/1

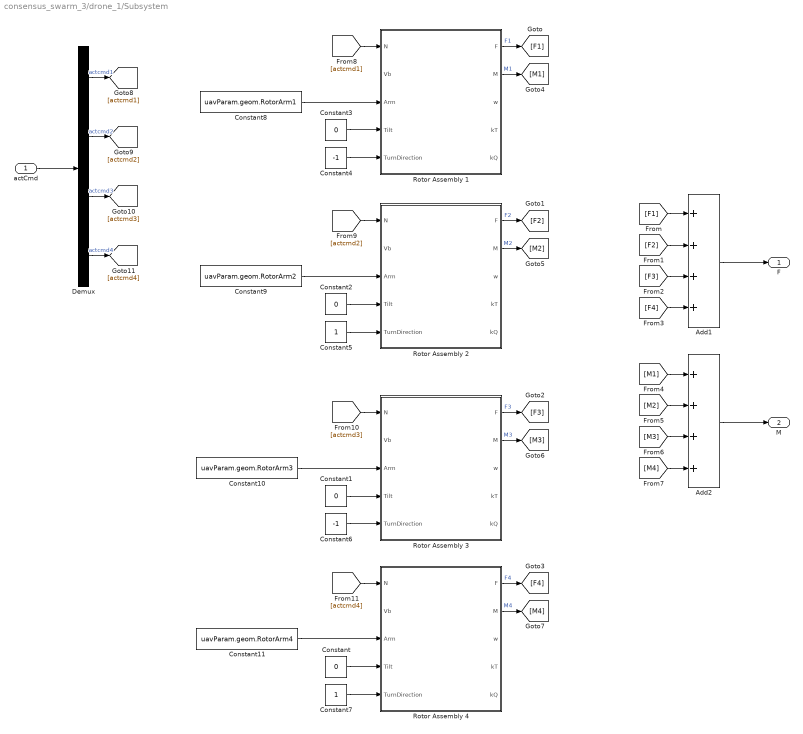
== system consensus_swarm_3/drone_1/Subsystem ==
  actCmd : Inport
  Add1 : Sum  Inputs=++++
  Add2 : Sum  Inputs=++++
  Constant{,1..3} (4 alike) : Constant  Value=0
  Constant10 : Constant  Value=uavParam.geom.RotorArm3
  Constant11 : Constant  Value=uavParam.geom.RotorArm4
  Constant4 : Constant  Value=-1
  Constant5 : Constant
  Constant6 : Constant  Value=-1
  Constant7 : Constant
  Constant8 : Constant  Value=uavParam.geom.RotorArm1
  Constant9 : Constant  Value=uavParam.geom.RotorArm2
  Demux : Demux
  Rotor Assembly 1 : Subsystem
  Rotor Assembly 2 : Subsystem
  Rotor Assembly 3 : Subsystem
  Rotor Assembly 4 : Subsystem
  F : Outport
  M : Outport  Port=2
  wires:
  [actcmd4] -> Rotor Assembly 4/1(N)
  Demux/4 -> [actcmd4]  "actcmd4"
  [actcmd3] -> Rotor Assembly 3/1(N)
  Demux/3 -> [actcmd3]  "actcmd3"
  [actcmd2] -> Rotor Assembly 2/1(N)
  Demux/2 -> [actcmd2]  "actcmd2"
  [actcmd1] -> Rotor Assembly 1/1(N)
  Demux/1 -> [actcmd1]  "actcmd1"
  actCmd/1 -> Demux/1
  [M4] -> Add2/4
  Rotor Assembly 4/2(M) -> [M4]  "M4"
  [M3] -> Add2/3
  Rotor Assembly 3/2(M) -> [M3]  "M3"
  [M2] -> Add2/2
  Rotor Assembly 2/2(M) -> [M2]  "M2"
  [M1] -> Add2/1
  Rotor Assembly 1/2(M) -> [M1]  "M1"
  [F4] -> Add1/4
  Rotor Assembly 4/1(F) -> [F4]  "F4"
  [F3] -> Add1/3
  Rotor Assembly 3/1(F) -> [F3]  "F3"
  [F2] -> Add1/2
  Rotor Assembly 2/1(F) -> [F2]  "F2"
  [F1] -> Add1/1
  Rotor Assembly 1/1(F) -> [F1]  "F1"
  Constant11/1 -> Rotor Assembly 4/3(Arm)
  Constant9/1 -> Rotor Assembly 2/3(Arm)
  Constant8/1 -> Rotor Assembly 1/3(Arm)
  Constant7/1 -> Rotor Assembly 4/5(TurnDirection)
  Constant5/1 -> Rotor Assembly 2/5(TurnDirection)
  Constant4/1 -> Rotor Assembly 1/5(TurnDirection)
  Constant3/1 -> Rotor Assembly 1/4(Tilt)
  Constant2/1 -> Rotor Assembly 2/4(Tilt)
  Constant/1 -> Rotor Assembly 4/4(Tilt)
  Add2/1 -> M/1
  Constant1/1 -> Rotor Assembly 3/4(Tilt)
  Constant6/1 -> Rotor Assembly 3/5(TurnDirection)
  ? -> Rotor Assembly 3/2(Vb)
  Add1/1 -> F/1
  Constant10/1 -> Rotor Assembly 3/3(Arm)
